simulink model "GROUNDHOOK"  (R2020b)
settings: Solver=VariableStepAuto  StartTime=0.0  StopTime=10  RelTol=1e-3
libraries: fl_lib x26, nesl_utility x9, sdl_lib x3, simulink x1
settings Model: Creator=kevin  LastModifiedBy=kevin

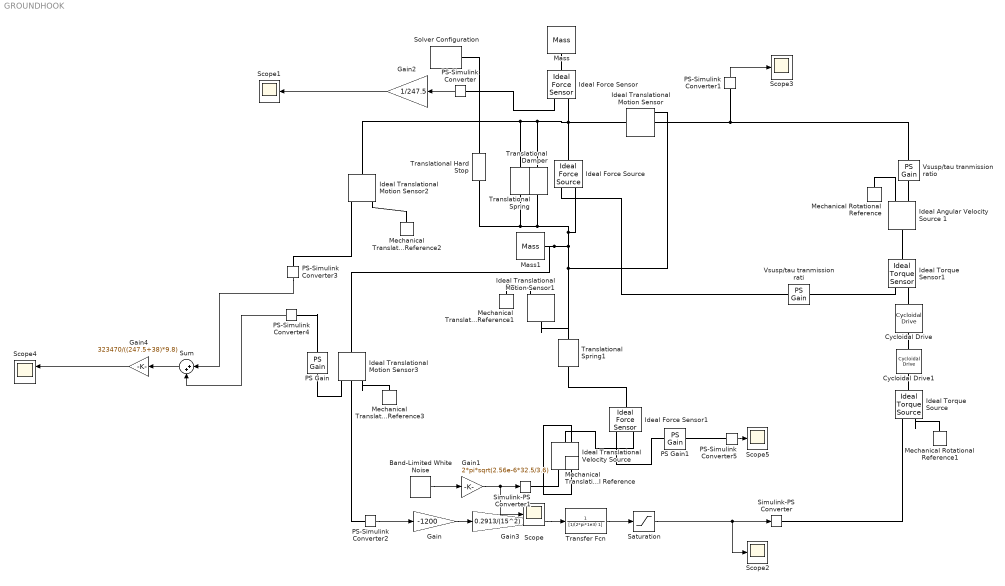
== system GROUNDHOOK ==
  Band-Limited White Noise : simulink/Sources/Band-Limited White Noise  Cov=[0.5]  Ts=0.001  seed=[23341]
  Cycloidal Drive : sdl_lib/Gears/Cycloidal Drive  n_cycloid=15  n_ring=16  friction_model=sdl.enum.gear_friction.none  eff_BF=0.90  eff_FB=0.05  temperature_TLU=[280, 300, 320] K  efficiency_BF_TLU=[.95, .85, .8]  efficiency_FB_TLU=[.1, .05, .03]  thermal_mass=50 J/K  pwr_thr=0.001 W  temperature_specify=off  temperature_priority=High  temperature=300 K  temperature_nominal_specify=off  temperature_nominal_unit=K  temperature_nominal_value=1
      settings: SourceProductBaseCode=LD  InternalSimscapePortConfiguration="{\"Bottom\":[],\"Left\":[{\"id\":\"B\",\"label\":\"B\",\"type\":\"foundation.mechanical.rotational.rotational\"}],\"Right\":[{\"id\":\"F\",\"label\":\"F\",\"type\":\"foundation.mechanical.rotational.rotational\"}],\"Top\":[]}"
  Cycloidal Drive1 : sdl_lib/Gears/Cycloidal Drive  n_cycloid=15  n_ring=16  friction_model=sdl.enum.gear_friction.none  eff_BF=0.90  eff_FB=0.05  temperature_TLU=[280, 300, 320] K  efficiency_BF_TLU=[.95, .85, .8]  efficiency_FB_TLU=[.1, .05, .03]  thermal_mass=50 J/K  pwr_thr=0.001 W  temperature_specify=off  temperature_priority=High  temperature=300 K  temperature_nominal_specify=off  temperature_nominal_unit=K  temperature_nominal_value=1
      settings: SourceProductBaseCode=LD  InternalSimscapePortConfiguration="{\"Bottom\":[],\"Left\":[{\"id\":\"B\",\"label\":\"B\",\"type\":\"foundation.mechanical.rotational.rotational\"}],\"Right\":[{\"id\":\"F\",\"label\":\"F\",\"type\":\"foundation.mechanical.rotational.rotational\"}],\"Top\":[]}"
  Gain : Gain  Gain=-1200
  Gain1 : Gain  Gain=2*pi*sqrt(2.56e-6*32.5/3.6)
  Gain2 : Gain  Gain=1/247.5
  Gain3 : Gain  Gain=0.2913/(15^2)
  Gain4 : Gain  Gain=323470/((247.5+38)*9.8)
  Ideal Angular Velocity Source 1 : fl_lib/Mechanical/Mechanical Sources/Ideal Angular Velocity Source
  Ideal Force Sensor : fl_lib/Mechanical/Mechanical Sensors/Ideal Force Sensor
  Ideal Force Sensor1 : fl_lib/Mechanical/Mechanical Sensors/Ideal Force Sensor
  Ideal Force Source : fl_lib/Mechanical/Mechanical Sources/Ideal Force Source
  Ideal Torque Sensor1 : fl_lib/Mechanical/Mechanical Sensors/Ideal Torque Sensor
  Ideal Torque Source : fl_lib/Mechanical/Mechanical Sources/Ideal Torque Source
  Ideal Translational Motion Sensor{,1..3} (4 alike) : fl_lib/Mechanical/Mechanical Sensors/Ideal Translational Motion Sensor  offset=0 m
  Ideal Translational Velocity Source : fl_lib/Mechanical/Mechanical Sources/Ideal Translational Velocity Source
  Mass : fl_lib/Mechanical/Translational Elements/Mass  mass=247.5 kg  num_ports=foundation.enum.numPorts2.one  v_specify=off  v_priority=High  v=0 m/s  v_nominal_specify=off  v_nominal_unit=m/s  v_nominal_value=1  f_specify=off  f_priority=None  f=0 N  f_nominal_specify=off  f_nominal_unit=N  f_nominal_value=1
  Mass1 : fl_lib/Mechanical/Translational Elements/Mass  mass=38 kg  num_ports=foundation.enum.numPorts2.one  v_specify=off  v_priority=High  v=0 m/s  v_nominal_specify=off  v_nominal_unit=m/s  v_nominal_value=1  f_specify=off  f_priority=None  f=0 N  f_nominal_specify=off  f_nominal_unit=N  f_nominal_value=1
  Mechanical Rotational Reference : fl_lib/Mechanical/Rotational Elements/Mechanical Rotational Reference
  Mechanical Rotational Reference1 : fl_lib/Mechanical/Rotational Elements/Mechanical Rotational Reference
  Mechanical Translational Reference{,1..3} (4 alike) : fl_lib/Mechanical/Translational Elements/Mechanical Translational Reference
  PS Gain : fl_lib/Physical Signals/Functions/PS Gain  gain=-1
  PS Gain1 : fl_lib/Physical Signals/Functions/PS Gain  gain=1/(247.5+38)/9.81
  PS-Simulink Converter{,1..5} (6 alike) : nesl_utility/PS-Simulink Converter  PhysicalDomain=network_engine_domain  SubClassName=ps_output  LeftPortType=input  RightPortType=output  PseudoPeriodic=off  Frequencies=[]  Unit=inherit  AffineConversion=off
  Saturation : Saturate  UpperLimit=2.27  LowerLimit=-2.27
  Scope{,1..3,5} (5 alike) : Scope
  Scope4 : Scope  NumInputPorts=2
  Simulink-PS Converter : nesl_utility/Simulink-PS Converter  PhysicalDomain=network_engine_domain  SubClassName=ps_input  LeftPortType=input  RightPortType=output  PseudoPeriodic=off  Frequencies=[]  NoiseDistribution=none  NoiseParameters=[]  Unit=1  AffineConversion=off  FilteringAndDerivatives=provide  SimscapeFilterOrder=1  InputFilterTimeConstant=0.001  UdotUserProvided=0
  Simulink-PS Converter1 : nesl_utility/Simulink-PS Converter  PhysicalDomain=network_engine_domain  SubClassName=ps_input  LeftPortType=input  RightPortType=output  PseudoPeriodic=off  Frequencies=[]  NoiseDistribution=none  NoiseParameters=[]  Unit=1  AffineConversion=off  FilteringAndDerivatives=provide  SimscapeFilterOrder=1  InputFilterTimeConstant=0.001  UdotUserProvided=0
  Solver Configuration : nesl_utility/Solver Configuration  PhysicalDomain=network_engine_domain  SubClassName=solver  LeftPortType=input  RightPortType=generic  Tones=[]  Harmonics=[]  SimulateNoise=off  Profile=off  UseLocalSampling=off  EnableSwitchedLinearOptims=on  FrequencyDomain=off  UseCCode=off  RelTol=0.001  AbsTol=1e-06  MinStep=1e-09  ToWorkspace=off  RevertToSquareIcSolve=off  NumHomotopyIterations=100  PhasorMode=off  PhasorModeNumHarmonics=1  DoDC=off  ResidualTolerance=1e-09  UseLocalSolver=off  LocalSolverChoice=NE_BACKWARD_EULER_ADVANCER  LocalSolverSampleTime=0.001  DoFixedCost=off  MaxNonlinIter=3  MaxModeIter=2  ComputeImpulses=off  ImpulseIterations=2  LinearAlgebra=auto  EquationFormulation=NE_TIME_EF  DelaysMemoryBudget=1024  AutomaticFiltering=on  FilteringTimeConstant=0.001  PartitionStorageMethod=AS_NEEDED  PartitionMemoryBudget=1024  PartitionMethod=ROBUST
  Sum : Sum  Inputs=|++
  Transfer Fcn : TransferFcn  Denominator=[1/(2*pi*1e3) 1]
  Translational Damper : sdl_lib/Couplings & Drives/Springs & Dampers/Translational Damper  D=800 N/(m/s)  enable_faults=0  b_fault=1e6 N/(m/s)  temporal_fault=0  fault_time=5 s  shock_fault=0  acceleration_limit=100 m/s^2  shock_limit=1  report_fault=1
      settings: SourceProductBaseCode=LD
  Translational Hard Stop : fl_lib/Mechanical/Translational Elements/Translational Hard Stop  upper_bnd=0.1 m  lower_bnd=-0.1 m  stiff_up=1e6 N/m  stiff_low=1e6 N/m  D_up=150 N/(m/s)  D_low=150 N/(m/s)  model=simscape.enum.hardstop.smooth  transition=0.1 mm  v_specify=off  v_priority=None  v=0 m/s  v_nominal_specify=off  v_nominal_unit=m/s  v_nominal_value=1  f_specify=off  f_priority=None  f=0 N  f_nominal_specify=off  f_nominal_unit=N  f_nominal_value=1  x_specify=on  x_priority=High  x=0 m  x_nominal_specify=off  x_nominal_unit=m  x_nominal_value=1
  Translational Spring : fl_lib/Mechanical/Translational Elements/Translational Spring  spr_rate=14070.1 N/m  v_specify=off  v_priority=None  v=0 m/s  v_nominal_specify=off  v_nominal_unit=m/s  v_nominal_value=1  f_specify=off  f_priority=None  f=0 N  f_nominal_specify=off  f_nominal_unit=N  f_nominal_value=1  x_specify=off  x_priority=High  x=0 m  x_nominal_specify=off  x_nominal_unit=m  x_nominal_value=1
  Translational Spring1 : fl_lib/Mechanical/Translational Elements/Translational Spring  spr_rate=323470 N/m  v_specify=off  v_priority=None  v=0 m/s  v_nominal_specify=off  v_nominal_unit=m/s  v_nominal_value=1  f_specify=off  f_priority=None  f=0 N  f_nominal_specify=off  f_nominal_unit=N  f_nominal_value=1  x_specify=off  x_priority=High  x=0 m  x_nominal_specify=off  x_nominal_unit=m  x_nominal_value=1
  Vsusp/tau tranmission rati : fl_lib/Physical Signals/Functions/PS Gain  gain=1/0.2913 rad/m
  Vsusp/tau tranmission ratio : fl_lib/Physical Signals/Functions/PS Gain  gain=1/0.2913 rad/m
  wires:
  Band-Limited White Noise/1 -> Gain1/1
  Gain1/1 -> Scope/1, Simulink-PS Converter1/1
  PS-Simulink Converter1/1 -> Scope3/1
  PS-Simulink Converter2/1 -> Gain/1
  Gain/1 -> Gain3/1
  PS-Simulink Converter/1 -> Gain2/1
  Transfer Fcn/1 -> Saturation/1
  Gain3/1 -> Transfer Fcn/1
  Saturation/1 -> Scope2/1, Simulink-PS Converter/1
  Gain2/1 -> Scope1/1
  Sum/1 -> Gain4/1
  PS-Simulink Converter4/1 -> Sum/2
  PS-Simulink Converter3/1 -> Sum/1
  Gain4/1 -> Scope4/1
  PS-Simulink Converter5/1 -> Scope5/1
  connections:
  Translational Spring/LConn1 -- Ideal Translational Motion Sensor2/LConn1 -- Translational Hard Stop/LConn1 -- Solver Configuration/RConn1 -- Translational Damper/LConn1 -- Ideal Force Source/LConn1 -- Ideal Force Sensor/RConn1 -- Ideal Translational Motion Sensor/LConn1
  Mass1/LConn1 -- Ideal Translational Motion Sensor3/LConn1 -- Ideal Translational Motion Sensor1/LConn1 -- Translational Spring1/LConn1 -- Ideal Translational Motion Sensor/RConn1 -- Ideal Force Source/RConn2 -- Translational Damper/RConn1 -- Translational Hard Stop/RConn1 -- Translational Spring/RConn1
  Mechanical Translational Reference/LConn1 -- Ideal Translational Velocity Source/RConn2
  Ideal Translational Motion Sensor/RConn2 -- PS-Simulink Converter1/LConn1 -- Vsusp/tau tranmission ratio/LConn1
  Simulink-PS Converter1/RConn1 -- Ideal Translational Velocity Source/RConn1
  Mechanical Rotational Reference/LConn1 -- Ideal Angular Velocity Source 1/RConn2
  Vsusp/tau tranmission ratio/RConn1 -- Ideal Angular Velocity Source 1/RConn1
  Cycloidal Drive/LConn1 -- Cycloidal Drive1/RConn1
  Ideal Torque Source/RConn2 -- Mechanical Rotational Reference1/LConn1
  Vsusp/tau tranmission rati/LConn1 -- Ideal Torque Sensor1/RConn2
  Ideal Torque Source/LConn1 -- Cycloidal Drive1/LConn1
  Mechanical Translational Reference1/LConn1 -- Ideal Translational Motion Sensor1/RConn1
  Mechanical Translational Reference2/LConn1 -- Ideal Translational Motion Sensor2/RConn1
  Ideal Translational Motion Sensor3/RConn1 -- Mechanical Translational Reference3/LConn1
  Ideal Torque Sensor1/RConn1 -- Cycloidal Drive/RConn1
  Ideal Angular Velocity Source 1/LConn1 -- Ideal Torque Sensor1/LConn1
  Vsusp/tau tranmission rati/RConn1 -- Ideal Force Source/RConn1
  Simulink-PS Converter/RConn1 -- Ideal Torque Source/RConn1
  PS-Simulink Converter/LConn1 -- Ideal Force Sensor/RConn2
  Mass/LConn1 -- Ideal Force Sensor/LConn1
  Ideal Translational Motion Sensor2/RConn3 -- PS-Simulink Converter3/LConn1
  Ideal Translational Motion Sensor3/RConn3 -- PS Gain/LConn1
  PS-Simulink Converter2/LConn1 -- Ideal Translational Motion Sensor3/RConn2
  PS Gain/RConn1 -- PS-Simulink Converter4/LConn1
  Ideal Translational Velocity Source/LConn1 -- Ideal Force Sensor1/RConn1
  Translational Spring1/RConn1 -- Ideal Force Sensor1/LConn1
  Ideal Force Sensor1/RConn2 -- PS Gain1/LConn1
  PS-Simulink Converter5/LConn1 -- PS Gain1/RConn1
